simulink model "Zad_3_szybkozmienny"  (R2018a)
settings: Solver=FixedStepAuto  StartTime=0.0  StopTime=0  RelTol=1e-3
libraries: CPOiS_SourcesSinks x6, CPOiS_DataManipulation x3, CPOiS_General x1
settings Model: Creator=rafal  LastModifiedBy=rafal

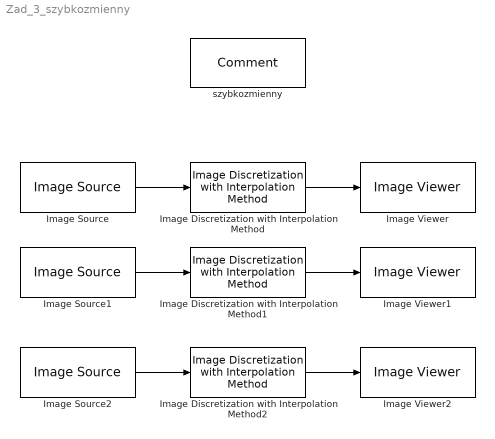
== system Zad_3_szybkozmienny ==
  Image Discretization with Interpolation Method : CPOiS_DataManipulation/Image Discretization with Interpolation Method  factor=4  method=nearest
      settings: SourceProductName=CPOiS - Digital image and signal processing
  Image Discretization with Interpolation Method1 : CPOiS_DataManipulation/Image Discretization with Interpolation Method  factor=4  method=bilinear
      settings: SourceProductName=CPOiS - Digital image and signal processing
  Image Discretization with Interpolation Method2 : CPOiS_DataManipulation/Image Discretization with Interpolation Method  factor=4  method=bicubic
      settings: SourceProductName=CPOiS - Digital image and signal processing
  Image Source : CPOiS_SourcesSinks/Image Source  FileSelection=gull.png
      settings: SourceProductName=CPOiS - Digital image and signal processing
  Image Source1 : CPOiS_SourcesSinks/Image Source  FileSelection=gull.png
      settings: SourceProductName=CPOiS - Digital image and signal processing
  Image Source2 : CPOiS_SourcesSinks/Image Source  FileSelection=gull.png
      settings: SourceProductName=CPOiS - Digital image and signal processing
  Image Viewer : CPOiS_SourcesSinks/Image Viewer
      settings: SourceProductName=CPOiS - Digital image and signal processing
  Image Viewer1 : CPOiS_SourcesSinks/Image Viewer
      settings: SourceProductName=CPOiS - Digital image and signal processing
  Image Viewer2 : CPOiS_SourcesSinks/Image Viewer
      settings: SourceProductName=CPOiS - Digital image and signal processing
  "szybkozmienny " : CPOiS_General/Comment
      settings: SourceProductName=CPOiS - Digital image and signal processing
  wires:
  Image Discretization with Interpolation Method2/1 -> Image Viewer2/1
  Image Source2/1 -> Image Discretization with Interpolation Method2/1
  Image Source/1 -> Image Discretization with Interpolation Method/1
  Image Source1/1 -> Image Discretization with Interpolation Method1/1
  Image Discretization with Interpolation Method1/1 -> Image Viewer1/1
  Image Discretization with Interpolation Method/1 -> Image Viewer/1
